simulink model "reverberation"  (R2021b)
settings: Solver=VariableStepAuto  StartTime=0.0  StopTime=1  RelTol=1e-3
libraries: dspsrcs4 x1
settings Model: Creator=holde  LastModifiedBy=Holden

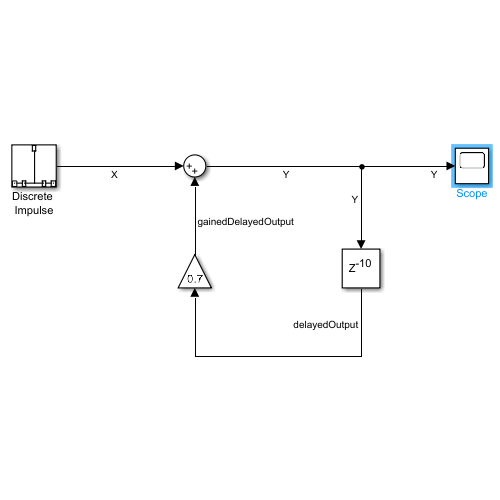
[thumbnail: Simulink's stored preview of the top-level diagram]
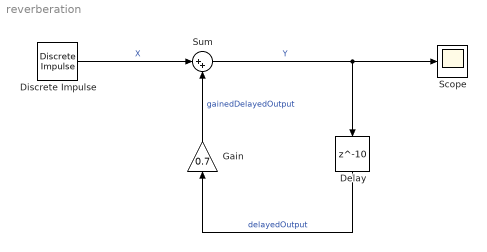
== system reverberation ==
  Delay : Delay  DelayLength=10  InitialCondition=0
  Discrete Impulse : dspsrcs4/Discrete  Impulse  Delay=0  SampleTime=1/48000  FrameSample=1  OutputFrames=off  dataType=double  isSigned=on  wordLen=16  udDataType=sfix(16)  fracBitsMode=Best precision  numFracBits=15  OutDataTypeStr=double  LastOutDataTypeStr=double
  Gain : Gain  Gain=0.7
  Scope : Scope
  Sum : Sum  Inputs=|++
  wires:
  Discrete Impulse/1 -> Sum/1  "X"
  Sum/1 -> Scope/1, Delay/1  "Y"
  Delay/1 -> Gain/1  "delayedOutput"
  Gain/1 -> Sum/2  "gainedDelayedOutput"
